simulink model "circuit"  (R2020b)
settings: Solver=FixedStepAuto  StartTime=0.0  StopTime=10  FixedStep=0.001  MaxStep=0.001  RelTol=1e-3
model workspace (MAT data in the model file):
  C = 10
  R = 10
settings Model: Creator=abhin  LastModifiedBy=abhin

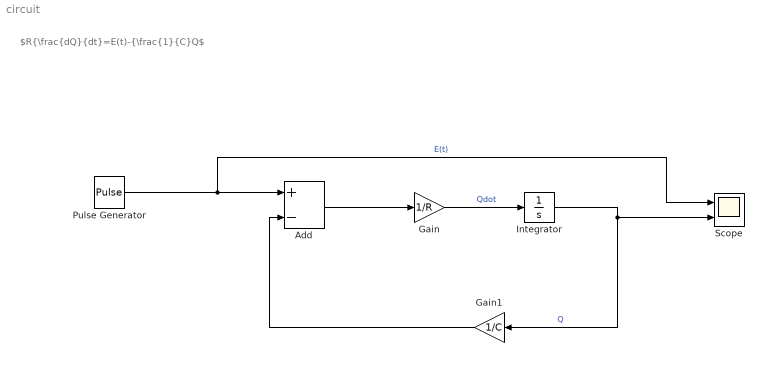
== system circuit ==
  note: $R{\frac{dQ}{dt}=E(t)-{\frac{1}{C}Q$
  Add : Sum  Inputs=+-
  Gain : Gain  Gain=1/R
  Gain1 : Gain  Gain=1/C
  Integrator : Integrator
  Pulse Generator : DiscretePulseGenerator  Amplitude=5
  Scope : Scope  NumInputPorts=2
  wires:
  Add/1 -> Gain/1
  Gain/1 -> Integrator/1  "Qdot"
  Integrator/1 -> Gain1/1, Scope/2  "Q"
  Pulse Generator/1 -> Scope/1, Add/1  "E(t)"
  Gain1/1 -> Add/2
